simulink model "Hz"  (R2020b)
settings: Solver=FixedStepDiscrete  StartTime=0.0  StopTime=N*dt  RelTol=1e-3
values from neighbouring files (symbols this model uses):
  dt = 1/Fs    (= 0.1)    [OverSmp.m]    (also in dsp_assist.m = 1e-06; signal_analysis.m = 0.001)
undefined symbols (not defined in the file or in its folder): a, vMix_int
libraries: dspsrcs4 x1
settings Model: Creator=User  LastModifiedBy=User

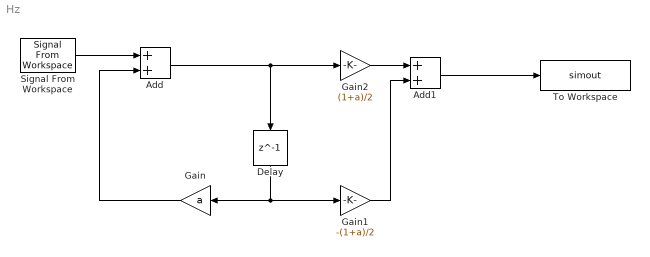
== system Hz ==
  Add : Sum
  Add1 : Sum
  Delay : Delay  DelayLength=1  SampleTime=dt
  Gain : Gain  Gain=a
  Gain1 : Gain  Gain=-(1+a)/2
  Gain2 : Gain  Gain=(1+a)/2
  Signal From Workspace : dspsrcs4/Signal From Workspace  X=abs(vMix_int)  Ts=dt  nsamps=1  OutputAfterFinalValue=Cyclic repetition  ignoreOrWarnInputAndFrameLengths=off  OutputFrames=off
  To Workspace : ToWorkspace  VariableName=simout  SampleTime=dt
      settings: Save2DSignal=2-D array (concatenate along first dimension)
  wires:
  Signal From Workspace/1 -> Add/1
  Add/1 -> Gain2/1, Delay/1
  Gain/1 -> Add/2
  Delay/1 -> Gain/1, Gain1/1
  Gain2/1 -> Add1/1
  Gain1/1 -> Add1/2
  Add1/1 -> To Workspace/1
